simulink model "offsetTest"  (R2016a)
settings: Solver=FixedStepAuto  StartTime=0.0  StopTime=inf  FixedStep=.01  RelTol=1e-3
libraries: aerolibanimutils x1, LibrarySimulinkSAS x1
settings Model: Creator=santd  LastModifiedBy=santd

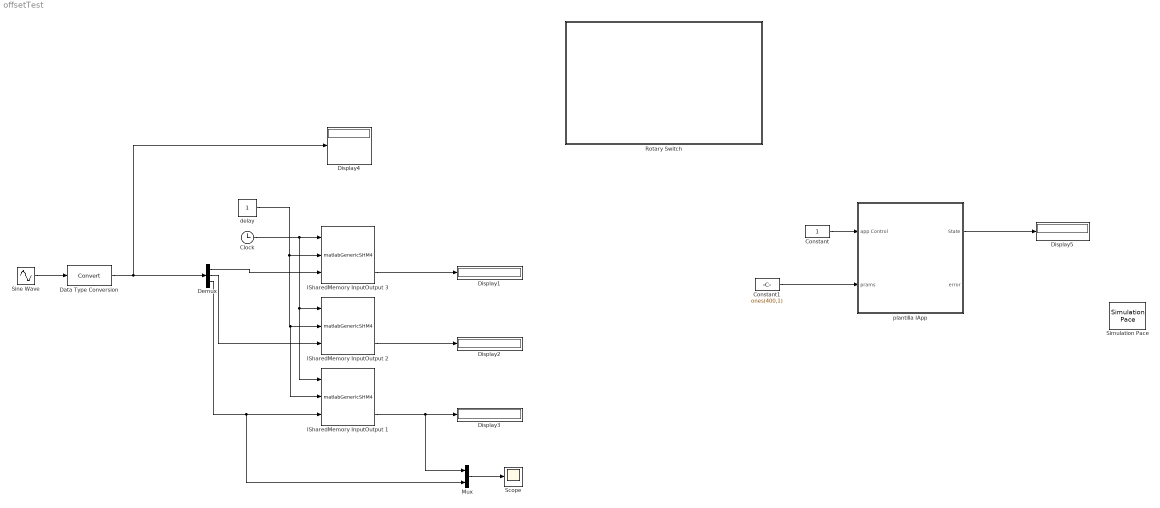
== system offsetTest ==
  Clock : Clock
  Constant : Constant
  Constant1 : Constant  Value=ones(400,1)
  Data Type Conversion : DataTypeConversion
  Demux : Demux  Outputs=3
  Display{1..5} (5 alike) : Display
  ISharedMemory InputOutput 1 : S-Function  FunctionName=matlabGenericSHM4  Parameters=nameIn,nameOut,vecE,vecS,tipoE,tipoS,ts,trigg,inOff,outOff  SFunctionDeploymentMode=off  EnableBusSupport=off  mask(Generic Share Memory block V2.0){nameIn='unimem_in', nameOut='unimem_out', vecE=[1 1 1], vecS=[1 1 1], tipoE=['d' 'd' 'f'], tipoS=['d' 'd' 'f'], ts=-1, inOff=40, outOff=40, trigg=off}
      mask prompts: nameIn "Input Shared Memory Name"; nameOut "Output Shared Memory Name"; vecE "Vector of system inputs"; vecS "Vector of system outputs"; tipoE "Data Types Inputs"; tipoS "Data Types Outputs"; ts "Sample Time"; inOff "Input Shared Memory Offset"; outOff "Output Shared Memory Offset"; trigg "Triggered writing"
      mask help:
      | This block allows Simulink communication with external processes through shared memory. It works on Unix and Windows.
      | More information in Help.
      mask Help:
      | Input Shared Memory Name: Name of the memory from which the physical device acquires its inputs.
      | Output Shared Memory Name: Name of the memory in which the physical device writes its output data.
      | Vector of system inputs: array that specify the number of inputs (array dimension) and the inputs size (array values)
      | Vector of system outputs: array that specify the number of outputs (array dimension) and the outputs size (array values)
      | Data types input: char array that specify each input types
      | Data types output: char array that specify each output types
      | Allowed types are:
      | ('f'=float, 'd'=double, 'i'=int32, 'c'=char, 'C'= unsigned char, 'I'=unsigned int)
      | 
      | Triggered writing: If trigger writing is selected, an additional block input is created at the end of inputs. When this input has a value greater than zero the data at the input of the block is written to the device input shared memory, otherwise the data is notwritten.
      | 
      | Example.
      | Suppose the following parameters:
      | Input Shared Memory Name = "devIn_1"
      | Output Shared Memory Name = "devOut_1"
      | Vector of system inputs=[3 2 1]
      | Vector of system outputs=[6 5 7 8]
      | Data types output=['f' 'I' 'c']
      | tipoS=['C' 'i' 'd' 'd']
      | 
      | Two Share Memories are created with names:
      | "devIn_1"(block input)
      | "devOut_1"  (block output)
      | 3 inputs are created:
      |  1° Dimension 3, type "unsigned char"
      |  2° Dimension 2, type "int"
      |  3° Dimension 1, type "char"
      | 4 outputs are created:
      |  1° Dimension 6, type "float"
      |  2° Dimension 5, type "unsigned int"
      |  3° Dimension 7, type "double"
      |  3° Dimension 8, type "double"
      mask Display: image('mem4.png')
  ISharedMemory InputOutput 2 : S-Function  FunctionName=matlabGenericSHM4  Parameters=nameIn,nameOut,vecE,vecS,tipoE,tipoS,ts,trigg,inOff,outOff  SFunctionDeploymentMode=off  EnableBusSupport=off  mask(Generic Share Memory block V2.0){nameIn='unimem_in', nameOut='unimem_out', vecE=[1 1 1], vecS=[1 1 1], tipoE=['d' 'd' 'f'], tipoS=['d' 'd' 'f'], ts=-1, inOff=20, outOff=20, trigg=off}
      mask prompts: nameIn "Input Shared Memory Name"; nameOut "Output Shared Memory Name"; vecE "Vector of system inputs"; vecS "Vector of system outputs"; tipoE "Data Types Inputs"; tipoS "Data Types Outputs"; ts "Sample Time"; inOff "Input Shared Memory Offset"; outOff "Output Shared Memory Offset"; trigg "Triggered writing"
      mask help:
      | This block allows Simulink communication with external processes through shared memory. It works on Unix and Windows.
      | More information in Help.
      mask Help:
      | Input Shared Memory Name: Name of the memory from which the physical device acquires its inputs.
      | Output Shared Memory Name: Name of the memory in which the physical device writes its output data.
      | Vector of system inputs: array that specify the number of inputs (array dimension) and the inputs size (array values)
      | Vector of system outputs: array that specify the number of outputs (array dimension) and the outputs size (array values)
      | Data types input: char array that specify each input types
      | Data types output: char array that specify each output types
      | Allowed types are:
      | ('f'=float, 'd'=double, 'i'=int32, 'c'=char, 'C'= unsigned char, 'I'=unsigned int)
      | 
      | Triggered writing: If trigger writing is selected, an additional block input is created at the end of inputs. When this input has a value greater than zero the data at the input of the block is written to the device input shared memory, otherwise the data is notwritten.
      | 
      | Example.
      | Suppose the following parameters:
      | Input Shared Memory Name = "devIn_1"
      | Output Shared Memory Name = "devOut_1"
      | Vector of system inputs=[3 2 1]
      | Vector of system outputs=[6 5 7 8]
      | Data types output=['f' 'I' 'c']
      | tipoS=['C' 'i' 'd' 'd']
      | 
      | Two Share Memories are created with names:
      | "devIn_1"(block input)
      | "devOut_1"  (block output)
      | 3 inputs are created:
      |  1° Dimension 3, type "unsigned char"
      |  2° Dimension 2, type "int"
      |  3° Dimension 1, type "char"
      | 4 outputs are created:
      |  1° Dimension 6, type "float"
      |  2° Dimension 5, type "unsigned int"
      |  3° Dimension 7, type "double"
      |  3° Dimension 8, type "double"
      mask Display: image('mem4.png')
  "ISharedMemory InputOutput 3 " : S-Function  FunctionName=matlabGenericSHM4  Parameters=nameIn,nameOut,vecE,vecS,tipoE,tipoS,ts,trigg,inOff,outOff  SFunctionDeploymentMode=off  EnableBusSupport=off  mask(Generic Share Memory block V2.0){nameIn='unimem_in', nameOut='unimem_out', vecE=[1 1 1], vecS=[1 1 1], tipoE=['d' 'd' 'f'], tipoS=['d' 'd' 'f'], ts=-1, inOff=0, outOff=0, trigg=off}
      mask prompts: nameIn "Input Shared Memory Name"; nameOut "Output Shared Memory Name"; vecE "Vector of system inputs"; vecS "Vector of system outputs"; tipoE "Data Types Inputs"; tipoS "Data Types Outputs"; ts "Sample Time"; inOff "Input Shared Memory Offset"; outOff "Output Shared Memory Offset"; trigg "Triggered writing"
      mask help:
      | This block allows Simulink communication with external processes through shared memory. It works on Unix and Windows.
      | More information in Help.
      mask Help:
      | Input Shared Memory Name: Name of the memory from which the physical device acquires its inputs.
      | Output Shared Memory Name: Name of the memory in which the physical device writes its output data.
      | Vector of system inputs: array that specify the number of inputs (array dimension) and the inputs size (array values)
      | Vector of system outputs: array that specify the number of outputs (array dimension) and the outputs size (array values)
      | Data types input: char array that specify each input types
      | Data types output: char array that specify each output types
      | Allowed types are:
      | ('f'=float, 'd'=double, 'i'=int32, 'c'=char, 'C'= unsigned char, 'I'=unsigned int)
      | 
      | Triggered writing: If trigger writing is selected, an additional block input is created at the end of inputs. When this input has a value greater than zero the data at the input of the block is written to the device input shared memory, otherwise the data is notwritten.
      | 
      | Example.
      | Suppose the following parameters:
      | Input Shared Memory Name = "devIn_1"
      | Output Shared Memory Name = "devOut_1"
      | Vector of system inputs=[3 2 1]
      | Vector of system outputs=[6 5 7 8]
      | Data types output=['f' 'I' 'c']
      | tipoS=['C' 'i' 'd' 'd']
      | 
      | Two Share Memories are created with names:
      | "devIn_1"(block input)
      | "devOut_1"  (block output)
      | 3 inputs are created:
      |  1° Dimension 3, type "unsigned char"
      |  2° Dimension 2, type "int"
      |  3° Dimension 1, type "char"
      | 4 outputs are created:
      |  1° Dimension 6, type "float"
      |  2° Dimension 5, type "unsigned int"
      |  3° Dimension 7, type "double"
      |  3° Dimension 8, type "double"
      mask Display: image('mem4.png')
  Mux : Mux  Inputs=2
  Rotary Switch : Subsystem  DialogController=hmiCreateDDGDialog  IsWebBlock=on  mask(MWDashboardBlock){webBlockId=34765018-ca77-4ea6-b429-27b5a5e2b0f2, webBlockType=discreteknob, ShowInLibBrowser=on, ShowInitialText=on, HMISrcModelName=offsetTest}
      mask prompts: webBlockId "WebBlock Id"; webBlockType "WebBlock Type"; HMISrcModelName "Source Model"
      mask Help: helpview([docroot '/mapfiles/simulink.map'], 'hmi_rotary_switch')
      mask Display:
      | model = bdroot(gcb);
      | if strcmp(get_param(model,'BlockDiagramType'), 'library')
      |     image([(matlabroot) '/toolbox/simulink/hmi/icons/DiscreteKnob.png']);
      | end
  Scope : Scope
  Simulation Pace : aerolibanimutils/Simulation Pace  SimulationPace=1  SleepMode=MATLAB Thread  OutputPaceError=off  SampleTime=-1
  Sine Wave : Sin  Amplitude=rand(3,1)  SampleTime=0
  delay : Constant
  plantilla IApp : Subsystem  mask{sys='IServer', shmControl='iServer_ctr', shmInput='unimem_in', shmOutput='unimem_out', shmInputVect=[60], shmOutputVect=[60], shmInputType=['C'], shmOutputType=['C'], period=100}
      mask prompts: sys "Program"; shmControl "Control Name"; shmInput "Input Name"; shmOutput "OutputName"; shmInputVect "Input Vector"; shmOutputVect "Output Vector"; shmInputType "Input Type"; shmOutputType "Output Type"; period "Period [us]"
      mask Display:
      | image('app.png')
      | color('blue');
      | port_label('input', 1, 'App Control')
      | port_label('input', 2, 'prams[char*]')
      | port_label('input', 3, 'Data In')
      | color('red');
      | port_label('output', 1, 'App ctr State')
      | port_label('output', 2, 'Error')
      | port_label('output', 3, 'Data Out')
  wires:
  Sine Wave/1 -> Data Type Conversion/1
  Data Type Conversion/1 -> Display4/1, Demux/1
  Clock/1 -> ISharedMemory InputOutput 1/1, ISharedMemory InputOutput 2/1, "ISharedMemory InputOutput 3 "/1
  delay/1 -> ISharedMemory InputOutput 1/2, ISharedMemory InputOutput 2/2, "ISharedMemory InputOutput 3 "/2
  Demux/1 -> "ISharedMemory InputOutput 3 "/3
  "ISharedMemory InputOutput 3 "/3 -> Display1/1
  ISharedMemory InputOutput 2/3 -> Display2/1
  ISharedMemory InputOutput 1/3 -> Mux/1, Display3/1
  Demux/2 -> ISharedMemory InputOutput 2/3
  Demux/3 -> Mux/2, ISharedMemory InputOutput 1/3
  Constant/1 -> plantilla IApp/1(app Control)
  Constant1/1 -> plantilla IApp/2(prams)
  plantilla IApp/1(State) -> Display5/1
  Mux/1 -> Scope/1

== system offsetTest/Rotary Switch ==

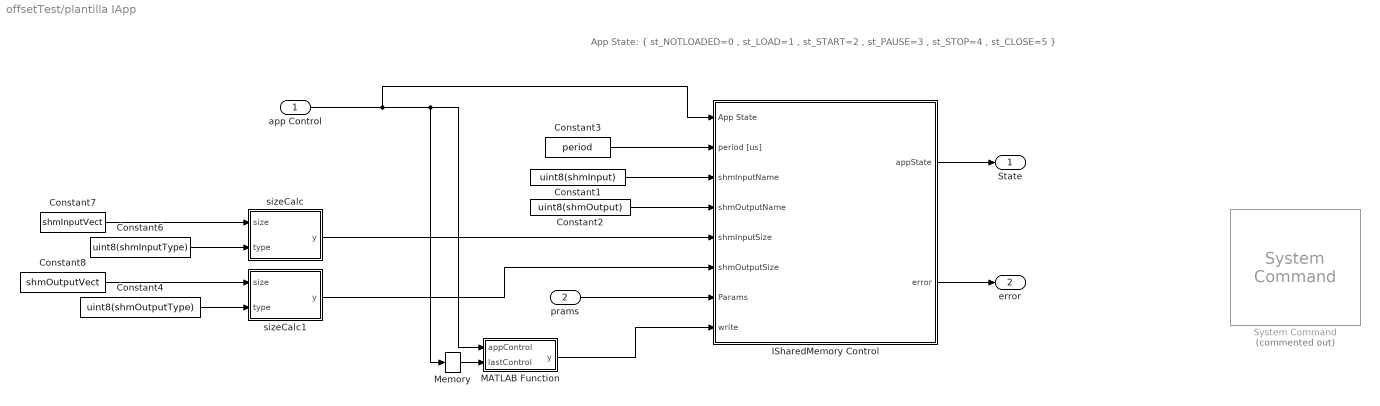
== system offsetTest/plantilla IApp ==
  note: App State: { st_NOTLOADED=0 , st_LOAD=1 , st_START=2 , st_PAUSE=3 , st_STOP=4 , st_CLOSE=5 }
  app Control : Inport
  prams : Inport  Port=2
  Constant1 : Constant  Value=uint8(shmInput)
  Constant2 : Constant  Value=uint8(shmOutput)
  Constant3 : Constant  Value=period
  Constant4 : Constant  Value=uint8(shmOutputType)  OutDataTypeStr=uint8
  Constant6 : Constant  Value=uint8(shmInputType)  OutDataTypeStr=uint8
  Constant7 : Constant  Value=shmInputVect
  Constant8 : Constant  Value=shmOutputVect
  ISharedMemory Control : Subsystem  mask{shmControl=shmControl}
      mask prompts: shmControl "Control Name"
      mask Display:
      | image('mem4.png')
      | color('blue');
      | port_label('input', 1, 'App Control')
      | port_label('input', 2, 'Period[us]')
      | port_label('input', 3, 'Input Name')
      | port_label('input', 4, 'Output Name')
      | port_label('input', 5, 'Input Size')
      | port_label('input', 6, 'Output Size')
      | port_label('input', 7, 'Prams')
      | port_label('input', 8, 'Write to mem')
      | color('red');
      | port_label('output', 1, 'App ctr State')
      | port_label('output', 2, 'Error')
  MATLAB Function : MATLAB Function  TreatAsAtomicUnit=on
  Memory : Memory  X0=25
  System Command : LibrarySimulinkSAS/System Command  Priority=0  Commented=on  start=' start SASDelay shmcontrol & timeout /t 10'  update=''  outputs=''  terminate='taskkill /IM SASDelay.exe'
  sizeCalc : MATLAB Function  TreatAsAtomicUnit=on
  sizeCalc1 : MATLAB Function  TreatAsAtomicUnit=on
  State : Outport
  error : Outport  Port=2
  wires:
  Constant4/1 -> sizeCalc1/2(type)
  Constant8/1 -> sizeCalc1/1(size)
  Constant6/1 -> sizeCalc/2(type)
  Constant7/1 -> sizeCalc/1(size)
  sizeCalc/1(y) -> ISharedMemory Control/5(shmInputSize)
  prams/1 -> ISharedMemory Control/7(Params)
  sizeCalc1/1(y) -> ISharedMemory Control/6(shmOutputSize)
  Memory/1 -> MATLAB Function/2(lastControl)
  Constant3/1 -> ISharedMemory Control/2(period [us])
  app Control/1 -> Memory/1, MATLAB Function/1(appControl), ISharedMemory Control/1(App State)
  ISharedMemory Control/1(appState) -> State/1
  ISharedMemory Control/2(error) -> error/1
  Constant1/1 -> ISharedMemory Control/3(shmInputName)
  Constant2/1 -> ISharedMemory Control/4(shmOutputName)
  MATLAB Function/1(y) -> ISharedMemory Control/8(write)

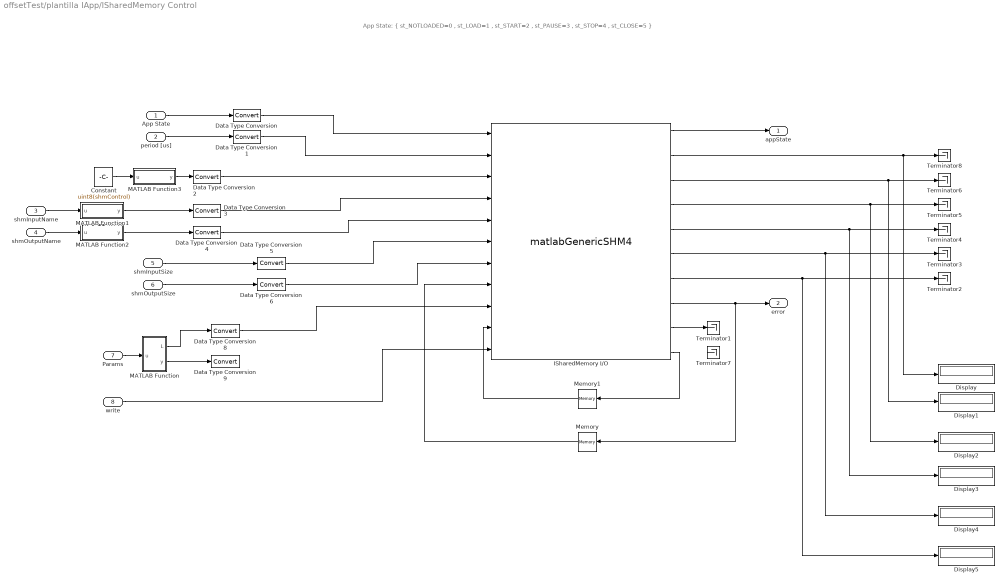
== system offsetTest/plantilla IApp/ISharedMemory Control ==
  note: App State: { st_NOTLOADED=0 , st_LOAD=1 , st_START=2 , st_PAUSE=3 , st_STOP=4 , st_CLOSE=5 }
  App State : Inport
  period [us] : Inport  Port=2
  shmInputName : Inport  Port=3
  shmOutputName : Inport  Port=4
  shmInputSize : Inport  Port=5
  shmOutputSize : Inport  Port=6
  Params : Inport  Port=7
  write : Inport  Port=8
  Constant : Constant  Value=uint8(shmControl)
  Data Type Conversion{,1..6,8..9} (9 alike) : DataTypeConversion
  Display{,1..5} (6 alike) : Display
  ISharedMemory I/O : S-Function  FunctionName=matlabGenericSHM4  Parameters=nameIn,nameOut,vecE,vecS,tipoE,tipoS,ts,trigg,inOff,outOff  SFunctionDeploymentMode=off  EnableBusSupport=off  mask(Generic Share Memory block V2.0){nameIn=shmControl, nameOut=shmControl, vecE=[1 1 40 40 40 1 1 1 1 400], vecS=[1 1 40 40 40 1 1 1 1 400], tipoE=['i' 'i' 'c' 'c' 'c' 'I' 'I' 'i' 'i' 'C'], tipoS=['i' 'i' 'c' 'c' 'c' 'I' 'I' 'i' 'i' 'C'], ts=-1, inOff=0, outOff=0, trigg=on}
      mask prompts: nameIn "Input Shared Memory Name"; nameOut "Output Shared Memory Name"; vecE "Vector of system inputs"; vecS "Vector of system outputs"; tipoE "Data Types Inputs"; tipoS "Data Types Outputs"; ts "Sample Time"; inOff "Input Shared Memory Offset"; outOff "Output Shared Memory Offset"; trigg "Triggered writing"
      mask help:
      | This block allows Simulink communication with external processes through shared memory. It works on Unix and Windows.
      | More information in Help.
      mask Help:
      | Input Shared Memory Name: Name of the memory from which the physical device acquires its inputs.
      | Output Shared Memory Name: Name of the memory in which the physical device writes its output data.
      | Vector of system inputs: array that specify the number of inputs (array dimension) and the inputs size (array values)
      | Vector of system outputs: array that specify the number of outputs (array dimension) and the outputs size (array values)
      | Data types input: char array that specify each input types
      | Data types output: char array that specify each output types
      | Allowed types are:
      | ('f'=float, 'd'=double, 'i'=int32, 'c'=char, 'C'= unsigned char, 'I'=unsigned int)
      | 
      | Triggered writing: If trigger writing is selected, an additional block input is created at the end of inputs. When this input has a value greater than zero the data at the input of the block is written to the device input shared memory, otherwise the data is notwritten.
      | 
      | Example.
      | Suppose the following parameters:
      | Input Shared Memory Name = "devIn_1"
      | Output Shared Memory Name = "devOut_1"
      | Vector of system inputs=[3 2 1]
      | Vector of system outputs=[6 5 7 8]
      | Data types output=['f' 'I' 'c']
      | tipoS=['C' 'i' 'd' 'd']
      | 
      | Two Share Memories are created with names:
      | "devIn_1"(block input)
      | "devOut_1"  (block output)
      | 3 inputs are created:
      |  1° Dimension 3, type "unsigned char"
      |  2° Dimension 2, type "int"
      |  3° Dimension 1, type "char"
      | 4 outputs are created:
      |  1° Dimension 6, type "float"
      |  2° Dimension 5, type "unsigned int"
      |  3° Dimension 7, type "double"
      |  3° Dimension 8, type "double"
      mask Display: image('mem4.png')
  MATLAB Function : MATLAB Function  TreatAsAtomicUnit=on
  MATLAB Function1 : MATLAB Function  TreatAsAtomicUnit=on
  MATLAB Function2 : MATLAB Function  TreatAsAtomicUnit=on
  MATLAB Function3 : MATLAB Function  TreatAsAtomicUnit=on
  Memory : Memory
  Memory1 : Memory
  Terminator{1..8} (8 alike) : Terminator
  appState : Outport
  error : Outport  Port=2
  wires:
  write/1 -> ISharedMemory I/O/11
  ISharedMemory I/O/2 -> Display/1, Terminator8/1
  ISharedMemory I/O/3 -> Display1/1, Terminator6/1
  ISharedMemory I/O/4 -> Display2/1, Terminator5/1
  ISharedMemory I/O/5 -> Display3/1, Terminator4/1
  ISharedMemory I/O/6 -> Display4/1, Terminator3/1
  ISharedMemory I/O/7 -> Display5/1, Terminator2/1
  ISharedMemory I/O/9 -> Terminator1/1
  Memory/1 -> ISharedMemory I/O/8
  ISharedMemory I/O/1 -> appState/1
  ISharedMemory I/O/8 -> error/1, Memory/1
  MATLAB Function/1(L) -> Data Type Conversion8/1
  Data Type Conversion2/1 -> ISharedMemory I/O/3
  MATLAB Function3/1(y) -> Data Type Conversion2/1
  MATLAB Function2/1(y) -> Data Type Conversion4/1
  MATLAB Function1/1(y) -> Data Type Conversion3/1
  MATLAB Function/2(y) -> Data Type Conversion9/1
  Constant/1 -> MATLAB Function3/1(u)
  Data Type Conversion8/1 -> ISharedMemory I/O/9
  Data Type Conversion6/1 -> ISharedMemory I/O/7
  Data Type Conversion5/1 -> ISharedMemory I/O/6
  Data Type Conversion4/1 -> ISharedMemory I/O/5
  Data Type Conversion3/1 -> ISharedMemory I/O/4
  Data Type Conversion1/1 -> ISharedMemory I/O/2
  Data Type Conversion/1 -> ISharedMemory I/O/1
  shmInputName/1 -> MATLAB Function1/1(u)
  shmInputSize/1 -> Data Type Conversion5/1
  shmOutputName/1 -> MATLAB Function2/1(u)
  shmOutputSize/1 -> Data Type Conversion6/1
  Params/1 -> MATLAB Function/1(u)
  App State/1 -> Data Type Conversion/1
  period [us]/1 -> Data Type Conversion1/1
  ISharedMemory I/O/10 -> Memory1/1
  Memory1/1 -> ISharedMemory I/O/10

== matlab function offsetTest/plantilla IApp/ISharedMemory Control/MATLAB Function ==
  data: L output; u input; y output
function [L,y] = fcn(u)
y=zeros(400,1);
L=length(u);
y(1:L,1)=u;

== matlab function offsetTest/plantilla IApp/ISharedMemory Control/MATLAB Function1 ==
  data: u input; y output
function y = fcn(u)
y=zeros(40,1);
y(1:length(u),1)=u;

== matlab function offsetTest/plantilla IApp/ISharedMemory Control/MATLAB Function2 ==
  data: u input; y output
function y = fcn(u)
y=zeros(40,1);
y(1:length(u),1)=u;

== matlab function offsetTest/plantilla IApp/ISharedMemory Control/MATLAB Function3 ==
  data: u input; y output
function y = fcn(u)
y=zeros(40,1);
y(1:length(u),1)=u;

== matlab function offsetTest/plantilla IApp/MATLAB Function ==
  data: appControl input; lastControl input; y output
function y = fcn(appControl,lastControl)
if(appControl~=lastControl)
    y=1;
else
    y=0;
end

== matlab function offsetTest/plantilla IApp/sizeCalc1 ==
  data: size input; y output; type input
function y = fcn(size,type)
n=length(size);
y=0;
for i=1:n
    switch type(i)
        case 'c'
            aux=size(i)*1;
        case 'C'
            aux=size(i)*1;
        case 'd'
            aux=size(i)*6;
        case 'f'
            aux=size(i)*4;
        case 'i'
            aux=size(i)*4;
        case 'I'
            aux=size(i)*4;
        otherwise %double
            aux=size(i)*6;
    end
y=y+aux;
end
end

== matlab function offsetTest/plantilla IApp/sizeCalc ==
  data: size input; y output; type input
function y = fcn(size,type)
n=length(size);
y=0;
for i=1:n
    switch type(i)
        case 'c'
            aux=size(i)*1;
        case 'C'
            aux=size(i)*1;
        case 'd'
            aux=size(i)*6;
        case 'f'
            aux=size(i)*4;
        case 'i'
            aux=size(i)*4;
        case 'I'
            aux=size(i)*4;
        otherwise %double
            aux=size(i)*6;
    end
y=y+aux;
end
end
